simulink model "Control_no_lineal_cartesiano"  (R2021a)
settings: Solver=VariableStepAuto  StartTime=0.0  StopTime=5  RelTol=1e-3
PreLoadFcn:
  | AUT_TP1_1;
InitFcn:
  | AUT_TP1_1;
undefined symbols (not defined in the file or in its folder): cfg
libraries: simulink x1
settings Model: Creator=Acer  LastModifiedBy=Acer

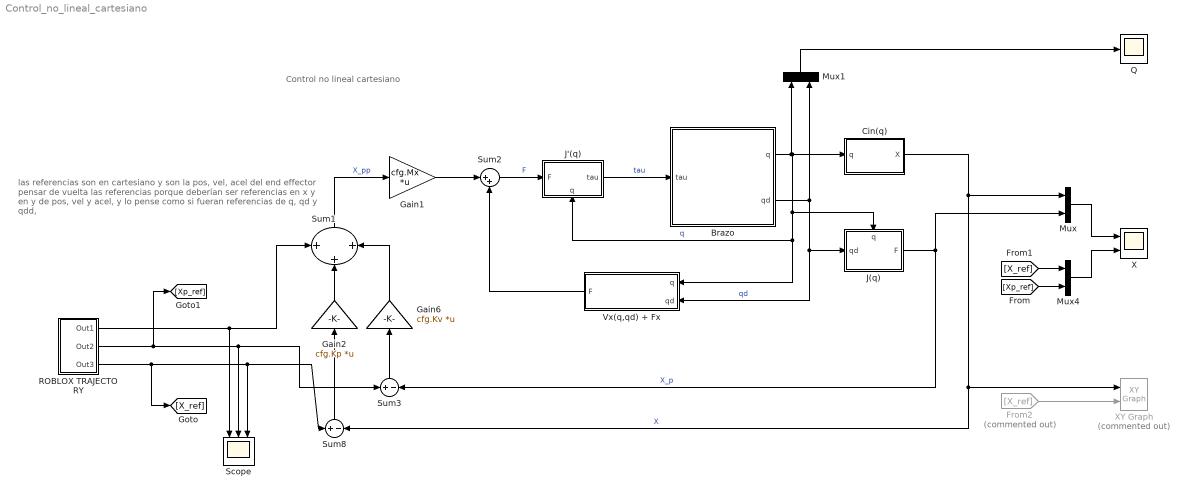
== system Control_no_lineal_cartesiano ==
  note: las referencias son en cartesiano
      | y son la pos, vel, acel del end effector
      |
      | pensar de vuelta las referencias porque deberían ser
      | referencias en x y en y de pos, vel y acel, y lo pense como si fueran
      | referencias de q, qd y qdd,
  note: Control no lineal cartesiano
  Brazo : Subsystem
      mask Display: image('$imagefile'); % Use "Edit Image" on toolstrip to change.
  Cin(q) : Subsystem
  From2 : From  Commented=on  GotoTag=X_ref  TagVisibility=global
  Gain1 : Gain  Gain=cfg.Mx  Multiplication=Matrix(K*u) (u vector)
  Gain2 : Gain  Gain=cfg.Kp  Multiplication=Matrix(K*u) (u vector)
  Gain6 : Gain  Gain=cfg.Kv  Multiplication=Matrix(K*u) (u vector)
  J'(q) : Subsystem
      settings: PortSchema="{\"entries\":[{\"content\":{\"sides\":[{\"content\":{\"connectorIds\":[\"In1\"]},\"type\":\"ConnectorPlacement.EquallySpacedRectSide\",\"uuid\":\"d38cc09c-49ff-41ee-9396-604e9f9ac0da\"},{\"content\":{\"connectorIds\":[\"Out1\"],\"side\":\"RIGHT\"},\"type\":\"ConnectorPlacement.EquallySpacedRectSide\",\"uuid\":\"131ff24e-374d-4df4-bf7f-b3f587a71233\"},{\"content\":{\"connectorIds\":[\"In2\"],\"side\":\"TOP\"},\"type\":\"ConnectorPlacement.EquallySpacedRectSide\",\"uuid\":\"57579f11-c71d-40a5-852c-e425271230cc\"},{\"content\":{\"connectorIds\":[],\"side\":\"BOTTOM\"},\"type\":\"ConnectorPlacement.EquallySpacedRectSide\",\"uuid\":\"61b5fd78-b202-42cc-a4f1-ea7da384d5e6\"}]},\"type\":\"ConnectorPlacement.EquallySpacedConnector\",\"uuid\":\"2fd97ed2-ef57-4ab9-8bdd-5bda36cd5779\"}],\"packageUris\":[\"http://schema.mathworks.com/mf0/Connector/R2020b\"],\"version\":\"1.0\"}"
  J(q) : Subsystem
      settings: PortSchema="{\"entries\":[{\"content\":{\"sides\":[{\"content\":{\"connectorIds\":[\"In1\"]},\"type\":\"ConnectorPlacement.EquallySpacedRectSide\",\"uuid\":\"d38cc09c-49ff-41ee-9396-604e9f9ac0da\"},{\"content\":{\"connectorIds\":[\"Out1\"],\"side\":\"RIGHT\"},\"type\":\"ConnectorPlacement.EquallySpacedRectSide\",\"uuid\":\"131ff24e-374d-4df4-bf7f-b3f587a71233\"},{\"content\":{\"connectorIds\":[\"In2\"],\"side\":\"TOP\"},\"type\":\"ConnectorPlacement.EquallySpacedRectSide\",\"uuid\":\"57579f11-c71d-40a5-852c-e425271230cc\"}]},\"type\":\"ConnectorPlacement.EquallySpacedConnector\",\"uuid\":\"2fd97ed2-ef57-4ab9-8bdd-5bda36cd5779\"}],\"packageUris\":[\"http://schema.mathworks.com/mf0/Connector/R2020b\"],\"version\":\"1.0\"}"
  Mux : Mux  Inputs=2
  Mux1 : Mux  Inputs=2
  Mux4 : Mux  Inputs=2
  Q : Scope
  ROBLOX TRAJECTORY : Subsystem
  Scope : Scope  NumInputPorts=3
  Sum1 : Sum  Inputs=+|+|+
  Sum2 : Sum  Inputs=|++
  Sum3 : Sum  Inputs=+-
  Sum8 : Sum  Inputs=+-
  Vx(q,qd) + Fx : Subsystem
  X : Scope  NumInputPorts=2
  XY Graph : simulink/Sinks/XY Graph  Commented=on  xmin=-1  xmax=1  ymin=-1  ymax=1  st=-1
  wires:
  Sum1/1 -> Gain1/1  "X_pp"
  Sum3/1 -> Gain6/1
  Sum8/1 -> Gain2/1
  Gain6/1 -> Sum1/3
  Gain1/1 -> Sum2/1
  Gain2/1 -> Sum1/2
  Sum2/1 -> J'(q)/1(F)  "F"
  J'(q)/1(tau) -> Brazo/1(tau)  "tau"
  Brazo/2(qd) -> Vx(q,qd) + Fx/2(qd), J(q)/1(qd), Mux1/2  "qd"
  J(q)/1(F) -> Sum3/2, Mux/2  "X_p"
  Cin(q)/1(X) -> Mux/1, XY Graph/1, Sum8/2  "X"
  Vx(q,qd) + Fx/1(F) -> Sum2/2
  Brazo/1(q) -> Cin(q)/1(q), Vx(q,qd) + Fx/1(q), J'(q)/2(q), J(q)/2(q), Mux1/1  "q"
  Mux/1 -> X/1
  Mux1/1 -> Q/1
  [Xp_ref] -> Mux4/2
  [X_ref] -> Mux4/1
  Mux4/1 -> X/2
  ROBLOX TRAJECTORY/3(Out3) -> [X_ref], Sum8/1, Scope/3
  ROBLOX TRAJECTORY/2(Out2) -> [Xp_ref], Sum3/1, Scope/2
  ROBLOX TRAJECTORY/1(Out1) -> Sum1/1, Scope/1
  From2/1 -> XY Graph/2

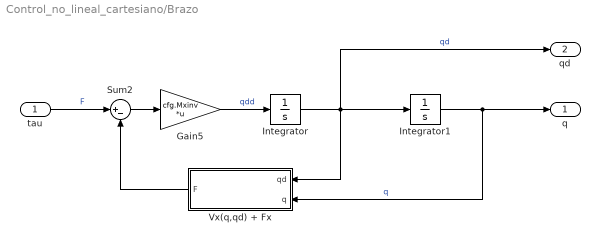
== system Control_no_lineal_cartesiano/Brazo ==
  tau : Inport
  Gain5 : Gain  Gain=cfg.Mxinv  Multiplication=Matrix(K*u) (u vector)
  Integrator : Integrator
  Integrator1 : Integrator  InitialCondition=5
  Sum2 : Sum  Inputs=|+-
  Vx(q,qd) + Fx : Subsystem
  q : Outport
  qd : Outport  Port=2
  wires:
  Gain5/1 -> Integrator/1  "qdd"
  Integrator/1 -> Vx(q,qd) + Fx/1(qd), Integrator1/1, qd/1  "qd"
  tau/1 -> Sum2/1  "F"
  Sum2/1 -> Gain5/1
  Integrator1/1 -> Vx(q,qd) + Fx/2(q), q/1  "q"
  Vx(q,qd) + Fx/1(F) -> Sum2/2

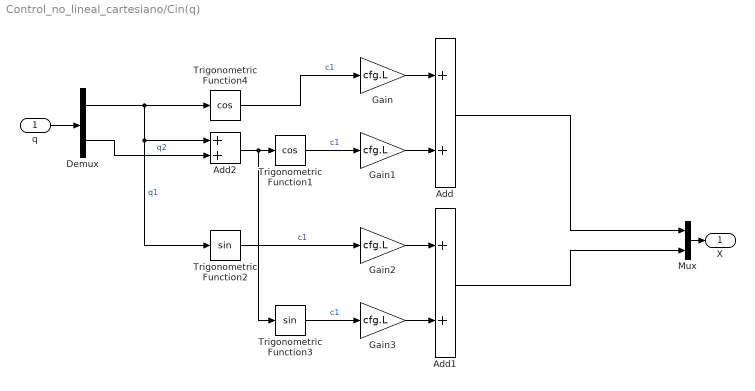
== system Control_no_lineal_cartesiano/Cin(q) ==
  q : Inport
  Add : Sum
  Add1 : Sum
  Add2 : Sum
  Demux : Demux  Outputs=2
  Gain{,1..3} (4 alike) : Gain  Gain=cfg.L
  Mux : Mux  Inputs=2
  Trigonometric Function1 : Trigonometry  Operator=cos
  Trigonometric Function2 : Trigonometry
  Trigonometric Function3 : Trigonometry
  Trigonometric Function4 : Trigonometry  Operator=cos
  X : Outport
  wires:
  Demux/1 -> Trigonometric Function2/1, Add2/1, Trigonometric Function4/1  "q1"
  q/1 -> Demux/1
  Mux/1 -> X/1
  Trigonometric Function4/1 -> Gain/1  "c1"
  Gain/1 -> Add/1
  Demux/2 -> Add2/2  "q2"
  Add2/1 -> Trigonometric Function3/1, Trigonometric Function1/1
  Trigonometric Function1/1 -> Gain1/1  "c1"
  Add/1 -> Mux/1
  Gain1/1 -> Add/2
  Trigonometric Function2/1 -> Gain2/1  "c1"
  Gain2/1 -> Add1/1
  Gain3/1 -> Add1/2
  Trigonometric Function3/1 -> Gain3/1  "c1"
  Add1/1 -> Mux/2

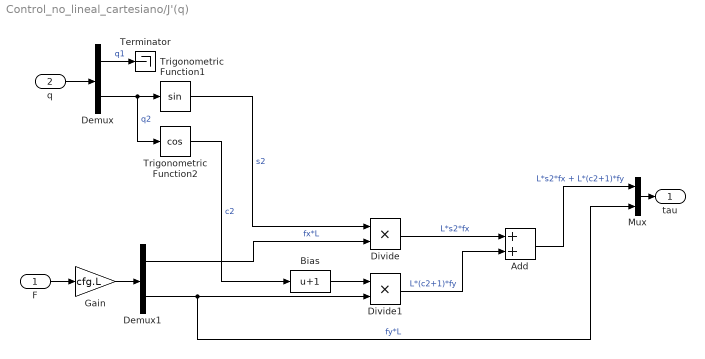
== system Control_no_lineal_cartesiano/J'(q) ==
  F : Inport
  q : Inport  Port=2
  Add : Sum
  Bias : Bias  Bias=1
  Demux : Demux  Outputs=2
  Demux1 : Demux  Outputs=2
  Divide : Product  Inputs=**
  Divide1 : Product  Inputs=**
  Gain : Gain  Gain=cfg.L
  Mux : Mux  Inputs=2
  Terminator : Terminator
  Trigonometric Function1 : Trigonometry
  Trigonometric Function2 : Trigonometry  Operator=cos
  tau : Outport
  wires:
  Demux/2 -> Trigonometric Function2/1, Trigonometric Function1/1  "q2"
  Demux/1 -> Terminator/1  "q1"
  q/1 -> Demux/1
  Trigonometric Function1/1 -> Divide/1  "s2"
  Trigonometric Function2/1 -> Bias/1  "c2"
  Demux1/1 -> Divide/2  "fx*L"
  Demux1/2 -> Mux/2, Divide1/2  "fy*L"
  Mux/1 -> tau/1
  F/1 -> Gain/1
  Gain/1 -> Demux1/1
  Divide/1 -> Add/1  "L*s2*fx"
  Bias/1 -> Divide1/1
  Divide1/1 -> Add/2  "L*(c2+1)*fy"
  Add/1 -> Mux/1  "L*s2*fx + L*(c2+1)*fy"

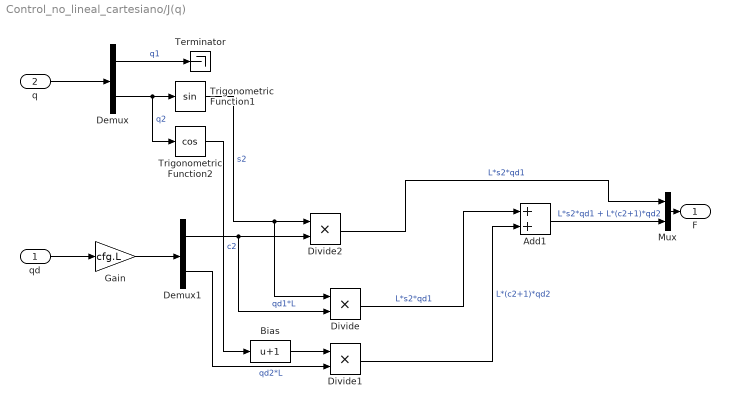
== system Control_no_lineal_cartesiano/J(q) ==
  qd : Inport
  q : Inport  Port=2
  Add1 : Sum
  Bias : Bias  Bias=1
  Demux : Demux  Outputs=2
  Demux1 : Demux  Outputs=2
  Divide : Product  Inputs=**
  Divide1 : Product  Inputs=**
  Divide2 : Product  Inputs=**
  Gain : Gain  Gain=cfg.L
  Mux : Mux  Inputs=2
  Terminator : Terminator
  Trigonometric Function1 : Trigonometry
  Trigonometric Function2 : Trigonometry  Operator=cos
  F : Outport
  wires:
  Divide1/1 -> Add1/2  "L*(c2+1)*qd2"
  Divide/1 -> Add1/1  "L*s2*qd1"
  q/1 -> Demux/1
  Bias/1 -> Divide1/1
  Demux/2 -> Trigonometric Function2/1, Trigonometric Function1/1  "q2"
  Gain/1 -> Demux1/1
  Mux/1 -> F/1
  Demux/1 -> Terminator/1  "q1"
  qd/1 -> Gain/1
  Add1/1 -> Mux/2  "L*s2*qd1 + L*(c2+1)*qd2"
  Demux1/1 -> Divide/2, Divide2/2  "qd1*L"
  Trigonometric Function1/1 -> Divide/1, Divide2/1  "s2"
  Divide2/1 -> Mux/1  "L*s2*qd1"
  Demux1/2 -> Divide1/2  "qd2*L"
  Trigonometric Function2/1 -> Bias/1  "c2"

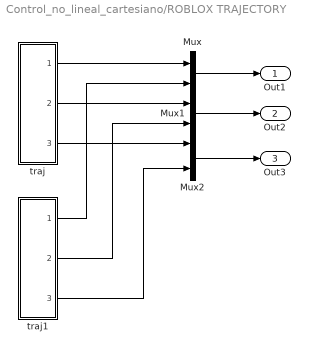
== system Control_no_lineal_cartesiano/ROBLOX TRAJECTORY ==
  Mux : Mux  Inputs=2
  Mux1 : Mux  Inputs=2
  Mux2 : Mux  Inputs=2
  traj : Subsystem
  traj1 : Subsystem
  Out1 : Outport
  Out2 : Outport  Port=2
  Out3 : Outport  Port=3
  wires:
  Mux/1 -> Out1/1
  Mux1/1 -> Out2/1
  Mux2/1 -> Out3/1
  traj/1(Out1) -> Mux/1
  traj/2(Out2) -> Mux1/1
  traj/3(Out3) -> Mux2/1
  traj1/1(Out1) -> Mux/2
  traj1/2(Out2) -> Mux1/2
  traj1/3(Out3) -> Mux2/2

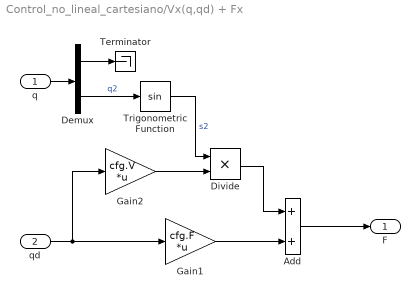
== system Control_no_lineal_cartesiano/Vx(q,qd) + Fx ==
  q : Inport
  qd : Inport  Port=2
  Add : Sum
  Demux : Demux  Outputs=2
  Divide : Product  Inputs=**
  Gain1 : Gain  Gain=cfg.F  Multiplication=Matrix(K*u) (u vector)
  Gain2 : Gain  Gain=cfg.V  Multiplication=Matrix(K*u) (u vector)
  Terminator : Terminator
  Trigonometric Function : Trigonometry
  F : Outport
  wires:
  qd/1 -> Gain1/1, Gain2/1
  Gain1/1 -> Add/2
  Add/1 -> F/1
  Gain2/1 -> Divide/2
  q/1 -> Demux/1
  Demux/1 -> Terminator/1
  Demux/2 -> Trigonometric Function/1  "q2"
  Divide/1 -> Add/1
  Trigonometric Function/1 -> Divide/1  "s2"

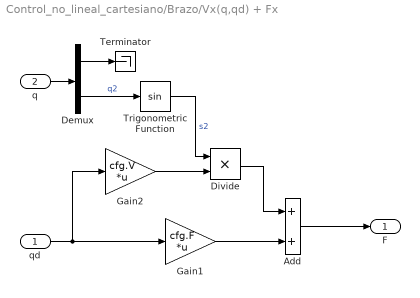
== system Control_no_lineal_cartesiano/Brazo/Vx(q,qd) + Fx ==
  qd : Inport
  q : Inport  Port=2
  Add : Sum
  Demux : Demux  Outputs=2
  Divide : Product  Inputs=**
  Gain1 : Gain  Gain=cfg.F  Multiplication=Matrix(K*u) (u vector)
  Gain2 : Gain  Gain=cfg.V  Multiplication=Matrix(K*u) (u vector)
  Terminator : Terminator
  Trigonometric Function : Trigonometry
  F : Outport
  wires:
  qd/1 -> Gain1/1, Gain2/1
  Gain1/1 -> Add/2
  Add/1 -> F/1
  Gain2/1 -> Divide/2
  q/1 -> Demux/1
  Demux/1 -> Terminator/1
  Demux/2 -> Trigonometric Function/1  "q2"
  Divide/1 -> Add/1
  Trigonometric Function/1 -> Divide/1  "s2"

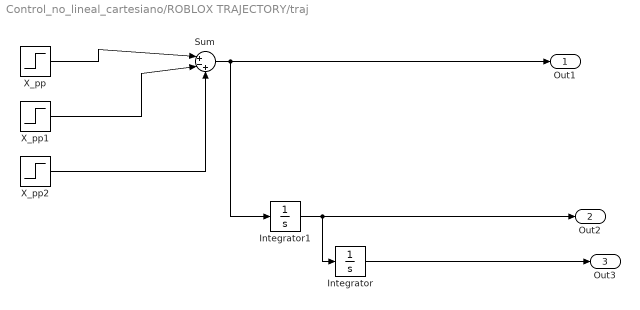
== system Control_no_lineal_cartesiano/ROBLOX TRAJECTORY/traj ==
  Integrator : Integrator
  Integrator1 : Integrator
  Sum : Sum  Inputs=|+-+
  X_pp : Step  Time=0.1  After=2  SampleTime=0
  X_pp1 : Step  After=4  SampleTime=0
  X_pp2 : Step  Time=1.9  After=2  SampleTime=0
  Out1 : Outport
  Out2 : Outport  Port=2
  Out3 : Outport  Port=3
  wires:
  X_pp/1 -> Sum/1
  Integrator1/1 -> Integrator/1, Out2/1
  Integrator/1 -> Out3/1
  X_pp1/1 -> Sum/2
  Sum/1 -> Out1/1, Integrator1/1
  X_pp2/1 -> Sum/3

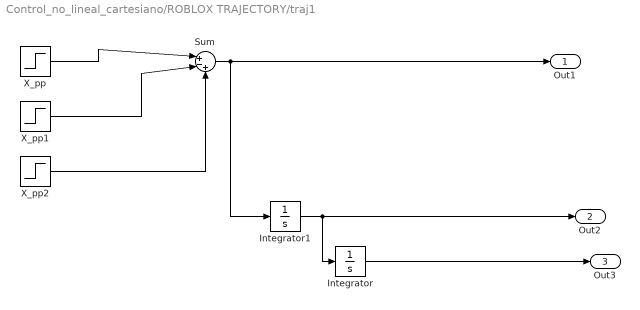
== system Control_no_lineal_cartesiano/ROBLOX TRAJECTORY/traj1 ==
  Integrator : Integrator
  Integrator1 : Integrator
  Sum : Sum  Inputs=|+-+
  X_pp : Step  Time=0.1  After=2  SampleTime=0
  X_pp1 : Step  After=4  SampleTime=0
  X_pp2 : Step  Time=1.9  After=2  SampleTime=0
  Out1 : Outport
  Out2 : Outport  Port=2
  Out3 : Outport  Port=3
  wires:
  X_pp/1 -> Sum/1
  Integrator1/1 -> Integrator/1, Out2/1
  Integrator/1 -> Out3/1
  X_pp1/1 -> Sum/2
  Sum/1 -> Out1/1, Integrator1/1
  X_pp2/1 -> Sum/3
